simulink model "water_tank_6th_feb_2023"  (R2022b)
settings: Solver=VariableStepAuto  StartTime=0.0  StopTime=t_end  RelTol=1e-3
undefined symbols (not defined in the file): A, A0, cd, g, h0, t_in, w_in_0, w_in_fin
settings Model: Creator=SMEA  LastModifiedBy=SMEA

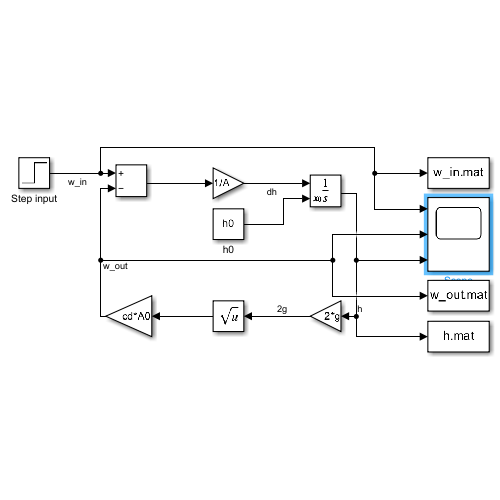
[thumbnail: Simulink's stored preview of the top-level diagram]
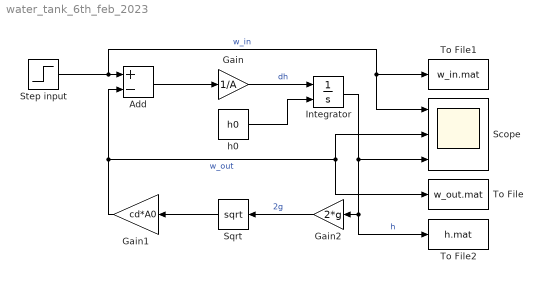
== system water_tank_6th_feb_2023 ==
  Add : Sum  Inputs=+-
  Gain : Gain  Gain=1/A
  Gain1 : Gain  Gain=cd*A0
  Gain2 : Gain  Gain=2*g
  Integrator : Integrator  InitialConditionSource=external
  Scope : Scope  NumInputPorts=3
  Sqrt : Sqrt
  Step input : Step  Time=t_in  Before=w_in_0  After=w_in_fin  SampleTime=0
  To File : ToFile  Filename=w_out.mat  SaveFormat=Timeseries
  To File1 : ToFile  Filename=w_in.mat  SaveFormat=Timeseries
  To File2 : ToFile  Filename=h.mat  SaveFormat=Timeseries
  h0 : Constant  Value=h0
  wires:
  Step input/1 -> Scope/1, To File1/1, Add/1  "w_in"
  Add/1 -> Gain/1
  Gain/1 -> Integrator/1  "dh"
  h0/1 -> Integrator/2
  Integrator/1 -> To File2/1, Gain2/1, Scope/3  "h"
  Gain2/1 -> Sqrt/1  "2g"
  Sqrt/1 -> Gain1/1
  Gain1/1 -> Add/2, To File/1, Scope/2  "w_out"
